simulink model "mainpoten"  (R2024b)
settings: Solver=FixedStepAuto  StartTime=0.0  StopTime=inf  RelTol=1e-3  EnableMultiTasking=on
libraries: stm32f4xxblockslib x2, dspstat3 x2
settings Model: STM32="{\"AnalogInput\":[{\"ID\":\"untitled:1\"},{\"ID\":\"main:1\"},{\"ID\":\"main:18\"},{\"ID\":\"mainpoten:18\"},{\"ID\":\"mainpoten:1\"}]}"  Creator=gamen  LastModifiedBy=gamen
settings OptimizationCC: DefaultParameterBehavior=Inlined  EnhancedBackFolding=on  PassReuseOutputArgsAs=Individual arguments  ZeroExternalMemoryAtStartup=off  ZeroInternalMemoryAtStartup=off  MaxStackSize=512  OptimizeBlockOrder=speed  DifferentSizesBufferReuse=on  OptimizationCustomize=off  EfficientTunableParamExpr=on
settings DebuggingCC: ParameterTunabilityLossMsg=error
settings HardwareCC: ProdBitPerPointer=32  ProdBitPerSizeT=32  ProdBitPerPtrDiffT=32  ProdLargestAtomicInteger=Long  ProdLargestAtomicFloat=Double  ProdWordSize=32  ProdLongLongMode=on  ProdHWDeviceType=ARM Compatible->ARM Cortex-M
settings SFSimCC: MATLABDynamicMemAlloc=off
settings RTWCC: Description=Embedded Coder  SystemTargetFile=ert.tlc  HardwareBoard=STM32G4xx Based  TemplateMakefile=ert_default_tmf  Toolchain=GNU Tools for ARM Embedded Processors
settings CodeAppCC: ForceParamTrailComments=on  IgnoreCustomStorageClasses=off  OperatorAnnotations=on  SimulinkDataObjDesc=on  SFDataObjDesc=on  InsertBlockDesc=on
settings ERTTargetCC: TargetLangStandard=C99 (ISO)  CodeReplacementLibrary=ARM Cortex-M  ExtModeTransport=3  ExtModeStaticAlloc=on  ExtModeStaticAllocSize=2048  ExtModeMexFile=ext_xcp  ExtModeIntrfLevel=Level2 - Open

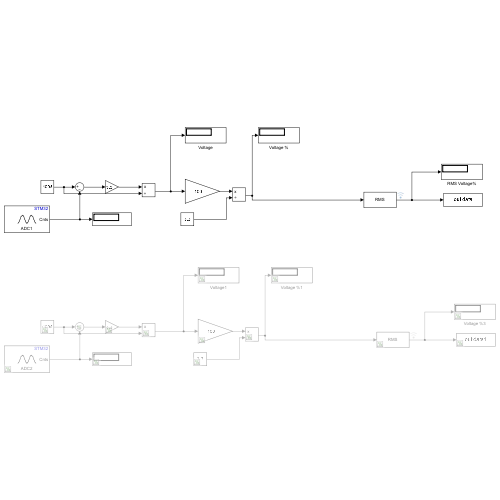
[thumbnail: Simulink's stored preview of the top-level diagram]
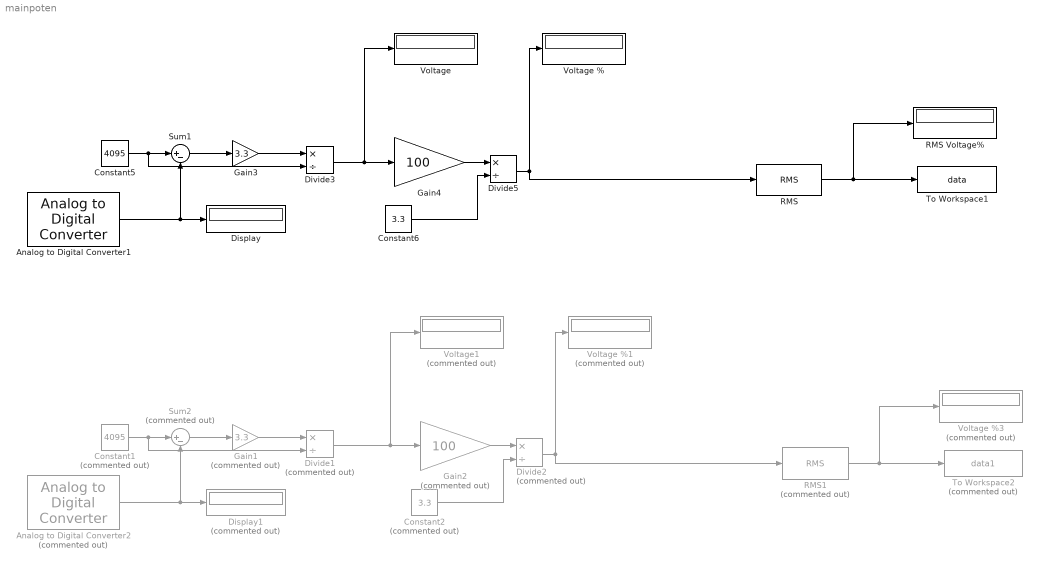
== system mainpoten ==
  Analog to Digital Converter1 : stm32f4xxblockslib/Analog to Digital Converter  ADCModule=ADC1  ConversionGroup=Regular  TriggerMode=Trigger and read  NumberOfConversions=1  EnableBufferConv=off  BufferLength=1  OutputStatus=off  SampleTime=-1  EnableSimPort=off  hoistedMaskSrc=ECSoC/ECSimCodegen/Analog to Digital Converter
  Analog to Digital Converter2 : stm32f4xxblockslib/Analog to Digital Converter  Commented=on  ADCModule=ADC2  ConversionGroup=Regular  TriggerMode=Trigger and read  NumberOfConversions=1  EnableBufferConv=off  BufferLength=1  OutputStatus=off  SampleTime=-1  EnableSimPort=off  hoistedMaskSrc=ECSoC/ECSimCodegen/Analog to Digital Converter
  Constant1 : Constant  Commented=on  Value=4095
  Constant2 : Constant  Commented=on  Value=3.3
  Constant5 : Constant  Value=4095
  Constant6 : Constant  Value=3.3
  Display : Display
  Display1 : Display  Commented=on
  Divide1 : Product  Commented=on  Inputs=*/
  Divide2 : Product  Commented=on  Inputs=*/
  Divide3 : Product  Inputs=*/
  Divide5 : Product  Inputs=*/
  Gain1 : Gain  Commented=on  Gain=3.3
  Gain2 : Gain  Commented=on  Gain=100
  Gain3 : Gain  Gain=3.3
  Gain4 : Gain  Gain=100
  RMS : dspstat3/RMS  run=off  directionMode=Each column  dimension=1  InputProcessing=Columns as channels (frame based)  reset_popup=None
  RMS Voltage% : Display
  RMS1 : dspstat3/RMS  Commented=on  run=off  directionMode=Each column  dimension=1  InputProcessing=Columns as channels (frame based)  reset_popup=None
  Sum1 : Sum  Inputs=|+-
  Sum2 : Sum  Commented=on  Inputs=|+-
  To Workspace1 : ToWorkspace  VariableName=data  SampleTime=-1
  To Workspace2 : ToWorkspace  Commented=on  VariableName=data1  SampleTime=-1
  Voltage : Display
  Voltage % : Display
  Voltage %1 : Display  Commented=on
  Voltage %3 : Display  Commented=on
  Voltage1 : Display  Commented=on
  wires:
  Gain3/1 -> Divide3/1
  Analog to Digital Converter1/1 -> Display/1, Sum1/2
  Divide3/1 -> Voltage/1, Gain4/1
  Gain4/1 -> Divide5/1
  Constant6/1 -> Divide5/2
  Sum1/1 -> Gain3/1
  Constant5/1 -> Sum1/1, Divide3/2
  Divide5/1 -> RMS/1, Voltage %/1
  RMS/1 -> RMS Voltage%/1, To Workspace1/1
  RMS1/1 -> Voltage %3/1, To Workspace2/1
  Divide2/1 -> RMS1/1, Voltage %1/1
  Sum2/1 -> Gain1/1
  Constant2/1 -> Divide2/2
  Gain2/1 -> Divide2/1
  Analog to Digital Converter2/1 -> Display1/1, Sum2/2
  Gain1/1 -> Divide1/1
  Divide1/1 -> Voltage1/1, Gain2/1
  Constant1/1 -> Sum2/1, Divide1/2
